simulink model "Ejer3_Prestamo"  (R2023b)
settings: Solver=FixedStepDiscrete  StartTime=0  StopTime=100  FixedStep=1  RelTol=1e-3
undefined symbols (not defined in the file): b0, c0, it
settings Model: Creator=alfre  LastModifiedBy=alfre

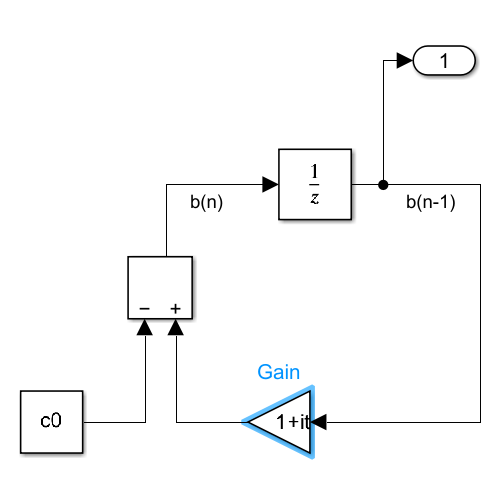
[thumbnail: Simulink's stored preview of the top-level diagram]
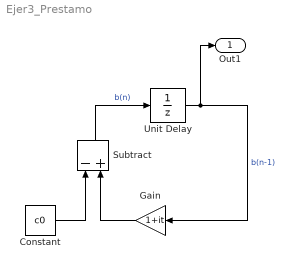
== system Ejer3_Prestamo ==
  Constant : Constant  Value=c0
  Gain : Gain  Gain=1+it
  Subtract : Sum  Inputs=-+
  Unit Delay : UnitDelay  InitialCondition=b0  SampleTime=-1  HasFrameUpgradeWarning=on
  Out1 : Outport
  wires:
  Unit Delay/1 -> Out1/1, Gain/1  "b(n-1)"
  Subtract/1 -> Unit Delay/1  "b(n)"
  Constant/1 -> Subtract/1
  Gain/1 -> Subtract/2
